simulink model "obsever"  (R2019b)
settings: Solver=VariableStepAuto  StartTime=0.0  StopTime=30  RelTol=1e-3
settings Model: Creator=63291  LastModifiedBy=63291

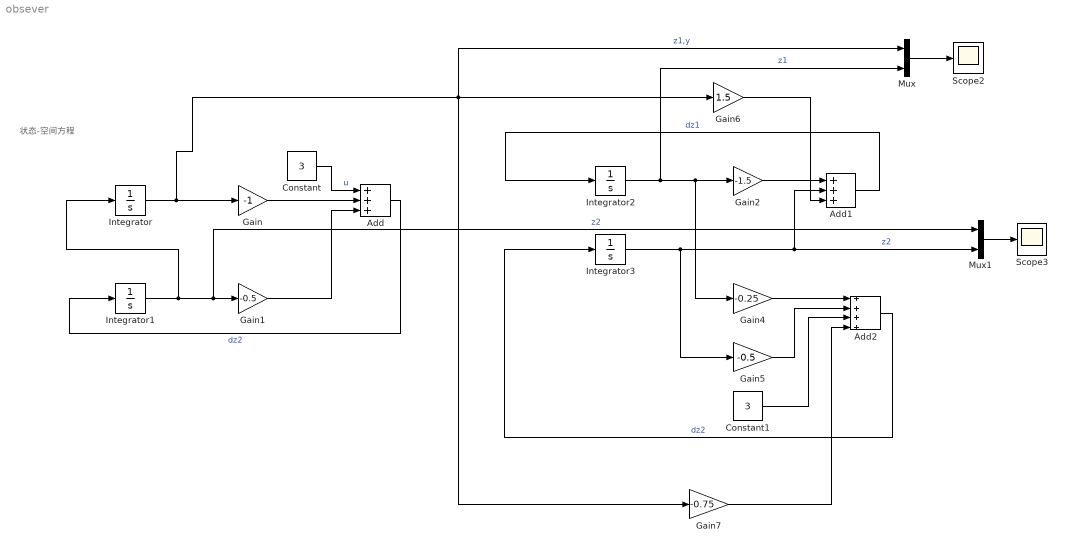
== system obsever ==
  note: 状态-空间方程
  Add : Sum  Inputs=+++
  Add1 : Sum  Inputs=+++
  Add2 : Sum  Inputs=++++
  Constant : Constant  Value=3
  Constant1 : Constant  Value=3
  Gain : Gain  Gain=-1
  Gain1 : Gain  Gain=-0.5
  Gain2 : Gain  Gain=-1.5
  Gain4 : Gain  Gain=-0.25
  Gain5 : Gain  Gain=-0.5
  Gain6 : Gain  Gain=1.5
  Gain7 : Gain  Gain=-0.75
  Integrator{,1..3} (4 alike) : Integrator
  Mux : Mux  Inputs=2
  Mux1 : Mux  Inputs=2
  Scope2 : Scope
  Scope3 : Scope
  wires:
  Integrator/1 -> Mux/1, Gain7/1, Gain6/1, Gain/1  "z1,y"
  Integrator1/1 -> Mux1/1, Gain1/1, Integrator/1  "z2"
  Add/1 -> Integrator1/1  "dz2"
  Constant/1 -> Add/1  "u"
  Gain1/1 -> Add/3
  Gain/1 -> Add/2
  Add1/1 -> Integrator2/1  "dz1"
  Integrator2/1 -> Mux/2, Gain4/1, Gain2/1  "z1"
  Add2/1 -> Integrator3/1  "dz2"
  Integrator3/1 -> Mux1/2, Add1/2, Gain5/1  "z2"
  Gain2/1 -> Add1/1
  Gain4/1 -> Add2/1
  Gain5/1 -> Add2/2
  Constant1/1 -> Add2/3
  Gain6/1 -> Add1/3
  Gain7/1 -> Add2/4
  Mux/1 -> Scope2/1
  Mux1/1 -> Scope3/1
